simulink model "local_agent"  (R2019a)
settings: Solver=VariableStepAuto  StartTime=0.0  StopTime=stopTime  RelTol=1e-3
undefined symbols (not defined in the file or in its folder): avg_usersArg, custom_action, lambda1Arg, lambda2Arg, lower_limitArg, random_seedArg, risk_delay_lengthArg, risk_delayArg, upper_limitArg
settings Model: Creator=ddavis  LastModifiedBy=Saurav

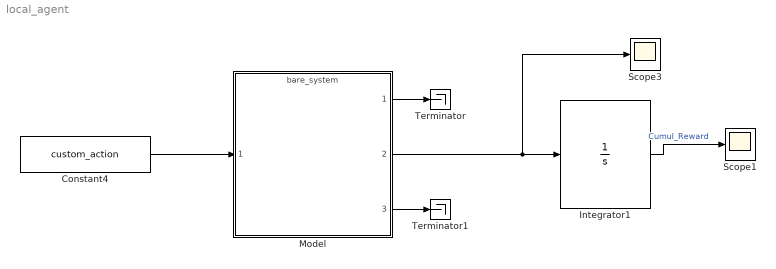
== system local_agent ==
  Constant4 : Constant  Value=custom_action
  Integrator1 : Integrator  ZeroCross=off
  Model : ModelReference  ModelNameDialog=bare_system  ParameterArgumentNames=lambda1Arg,lambda2Arg,random_seedArg,avg_usersArg,risk_delayArg,risk_delay_lengthArg,lower_limitArg,upper_limitArg  ParameterArgumentValues=7,1,5,3,1,0,50,100  UsingDefaultArgumentValue=0,0,0,0,0,0,0,0  SimulationMode=Normal  ModelReferenceVersion=1.146
  Scope1 : Scope
  Scope3 : Scope
  Terminator : Terminator
  Terminator1 : Terminator
  wires:
  Model/2 -> Scope3/1, Integrator1/1
  Integrator1/1 -> Scope1/1  "Cumul_Reward"
  Model/1 -> Terminator/1
  Model/3 -> Terminator1/1
  Constant4/1 -> Model/1
